simulink library "halout"  (R2021b)
settings: Solver=VariableStepAuto  StartTime=0.0  StopTime=10.0  RelTol=1e-3
undefined symbols (not defined in the file): C_TASK_5MS_S, FALSE, KHAL_CAN1FD1APS3E2E_flg, KHAL_CAN1FD1APS3TxReq_flg, KHAL_CAN1FD1VCU2E2E_flg, KHAL_CAN1FD1VCU2TxReq_flg, KHAL_CAN1FD1VCU3E2E_flg, KHAL_CAN1FD1VCU3TxReq_flg, KHAL_CAN1TxReq_flg, KHAL_CAN1VMCFCM1E2E_flg, KHAL_CAN1VMCFCM1TxReq_flg, KHAL_CAN2TxReq_flg, KHAL_CAN3FD3VCU1toNIDECTxReq_flg, KHAL_CAN3FD3VCU1TxReq_flg, KHAL_CAN3FD3VCU2E2E_flg, KHAL_CAN3FD3VCU2toNIDECE2E_flg, KHAL_CAN3FD3VCU2toNIDECTxReq_flg, KHAL_CAN3FD3VCU2TxReq_flg, KHAL_CAN3TxReq_flg, KHAL_CAN4FD4CE1000E2E_flg, KHAL_CAN4FD4CE1000TxReq_flg, KHAL_CAN4TxReq_flg, KHAL_CAN5TxReq_flg, KHAL_CAN6FD6APS3E2E_flg, KHAL_CAN6FD6APS3TxReq_flg, KHAL_CAN6FD6VCU2E2E_flg, KHAL_CAN6FD6VCU2TxReq_flg, KHAL_CAN6TxReq_flg, ONE_INT, TRUE, ZERO_INT
libraries: FVT_lib x549, simulink x244
(part 27 of 27)

== matlab function halout/HAL_OUT/CAN6/FD6_APS3_0x238/CRC8_IfAction_Tx/If Action Subsystem/CRC8_Caculation/MATLAB Function ==
  data: msg_raw input; CRC_Out output
function CRC_Out= fcn(msg_raw)

divisor = 0x1D;
messageLength = 8;
CRC_raw = uint8(0xFF);

for i = 1:length(msg_raw(:,1))

    message = bitxor(CRC_raw,msg_raw(i));

    for k = 1:messageLength
        if bitget(message,8)
            message = bitshift(message,1);
            message = bitxor(message,divisor);
        else
            message = bitshift(message,1);
        end
    end
    CRC_raw = message;

end

CRC_Out = bitxor(CRC_raw,0xFF);

== matlab function halout/HAL_OUT/CAN6/FD6_APS3_0x238/CRC8_IfAction_Tx/If Action Subsystem1/CRC8_E2EProfile1/MATLAB Function ==
  data: msg_raw input; CRC_Out output
function CRC_Out= fcn(msg_raw)

divisor = 0x1D;
messageLength = 8;
CRC_raw = uint8(0x00);

for i = 1:length(msg_raw(:,1))

    message = bitxor(CRC_raw,msg_raw(i));

    for k = 1:messageLength
        if bitget(message,8)
            message = bitshift(message,1);
            message = bitxor(message,divisor);
        else
            message = bitshift(message,1);
        end
    end
    CRC_raw = message;

end

CRC_Out = bitxor(CRC_raw,0x00);

== stateflow chart halout/HAL_OUT/CAN6/FD6_VCU2_Tx/Chart ==
  state TrigCounter
    en:
    counter = 0;
    counter++;
    (default) -> (junction 5)
    TrigCounter -> (junction 5) : {
        | counter++;
        | }
    (junction 5) -> (junction 6) [order 1] : [TxReq && (counter %% CycleCnt) == 0]
    (junction 5) -> (junction 7) [order 2]
    (junction 6) -> (junction 8) : {
        | TxTrigger;
        | counter = 0;
        | }
    (junction 8) -> (junction 7)
    (junction 7) -> (junction 34)
    (junction 34) -> (junction 33) [order 1] : [ !TxReq]
    (junction 34) -> (junction 35) [order 2]
    (junction 33) -> (junction 36) : {
        | counter = 0;
        | }
    (junction 36) -> (junction 35)
    (junction 35) -> (junction 44)
  data: TxReq input; CycleCnt input; counter local uint16
  events: TxTrigger output FUNCTION_CALL_EVENT

== matlab function halout/HAL_OUT/CAN6/FD6_VCU2_0x154/CRC8_IfAction_Tx/If Action Subsystem/CRC8_Caculation/MATLAB Function ==
  data: msg_raw input; CRC_Out output
function CRC_Out= fcn(msg_raw)

divisor = 0x1D;
messageLength = 8;
CRC_raw = uint8(0xFF);

for i = 1:length(msg_raw(:,1))

    message = bitxor(CRC_raw,msg_raw(i));

    for k = 1:messageLength
        if bitget(message,8)
            message = bitshift(message,1);
            message = bitxor(message,divisor);
        else
            message = bitshift(message,1);
        end
    end
    CRC_raw = message;

end

CRC_Out = bitxor(CRC_raw,0xFF);

== matlab function halout/HAL_OUT/CAN6/FD6_VCU2_0x154/CRC8_IfAction_Tx/If Action Subsystem1/CRC8_E2EProfile1/MATLAB Function ==
  data: msg_raw input; CRC_Out output
function CRC_Out= fcn(msg_raw)

divisor = 0x1D;
messageLength = 8;
CRC_raw = uint8(0x00);

for i = 1:length(msg_raw(:,1))

    message = bitxor(CRC_raw,msg_raw(i));

    for k = 1:messageLength
        if bitget(message,8)
            message = bitshift(message,1);
            message = bitxor(message,divisor);
        else
            message = bitshift(message,1);
        end
    end
    CRC_raw = message;

end

CRC_Out = bitxor(CRC_raw,0x00);

== stateflow chart halout/HAL_OUT/CAN_Scheduler ==
  state CAN_scheduler
    (default) -> (junction 55)
    CAN_scheduler -> (junction 55)
    (junction 55) -> (junction 53) [order 1] : [KHAL_CAN1TxReq_flg && VOUTP_ALLCANTxReq_flg]
    (junction 55) -> (junction 214) [order 2]
    (junction 53) -> (junction 212) : {
        | trig_can1;
        | }
    (junction 212) -> (junction 214)
    (junction 214) -> (junction 250)
    (junction 250) -> (junction 251) [order 1] : [KHAL_CAN2TxReq_flg && VOUTP_ALLCANTxReq_flg]
    (junction 250) -> (junction 253) [order 2]
    (junction 251) -> (junction 247) : {
        | trig_can2;
        | }
    (junction 247) -> (junction 253)
    (junction 253) -> (junction 258)
    (junction 258) -> (junction 259) [order 1] : [KHAL_CAN3TxReq_flg && VOUTP_ALLCANTxReq_flg]
    (junction 258) -> (junction 261) [order 2]
    (junction 259) -> (junction 255) : {
        | trig_can3;
        | }
    (junction 255) -> (junction 261)
    (junction 261) -> (junction 266)
    (junction 266) -> (junction 267) [order 1] : [KHAL_CAN4TxReq_flg && VOUTP_ALLCANTxReq_flg]
    (junction 266) -> (junction 269) [order 2]
    (junction 267) -> (junction 263) : {
        | trig_can4;
        | }
    (junction 263) -> (junction 269)
    (junction 269) -> (junction 274)
    (junction 274) -> (junction 275) [order 1] : [KHAL_CAN5TxReq_flg && VOUTP_ALLCANTxReq_flg]
    (junction 274) -> (junction 277) [order 2]
    (junction 275) -> (junction 271) : {
        | trig_can5;
        | }
    (junction 271) -> (junction 277)
    (junction 277) -> (junction 323)
    (junction 323) -> (junction 322) [order 1] : [KHAL_CAN6TxReq_flg && VOUTP_ALLCANTxReq_flg]
    (junction 323) -> (junction 324) [order 2]
    (junction 322) -> (junction 321) : {
        | trig_can6;
        | }
    (junction 321) -> (junction 324)
  data: KHAL_CAN1TxReq_flg input; KHAL_CAN2TxReq_flg input; KHAL_CAN3TxReq_flg input; KHAL_CAN4TxReq_flg input; KHAL_CAN5TxReq_flg input; KHAL_CAN6TxReq_flg input; VOUTP_ALLCANTxReq_flg input
  events: trig_can1 output FUNCTION_CALL_EVENT; trig_can2 output FUNCTION_CALL_EVENT; trig_can3 output FUNCTION_CALL_EVENT; trig_can4 output FUNCTION_CALL_EVENT; trig_can5 output FUNCTION_CALL_EVENT; trig_can6 output FUNCTION_CALL_EVENT
